simulink model "MCU_Input"  (R2022b)
settings: Solver=FixedStepDiscrete  StartTime=0.0  StopTime=10.0  FixedStep=1e-4  RelTol=1e-3
values from neighbouring files (symbols this model uses):
  C_ADC_Acc1Offset_i32 = 0.0    [MCU_Input_Sldd.sldd]    (also in MCU_Input_Sldd_objects.m = myPackage.Parameter)
  C_ADC_BrakeOffset_i32 = 0.0    [MCU_Input_Sldd.sldd]    (also in MCU_Input_Sldd_objects.m = myPackage.Parameter)
  C_ADC_HSTempGain_f32 = 0.0    [MCU_Input_Sldd.sldd]    (also in MCU_Input_Sldd_objects.m = myPackage.Parameter)
  C_ADC_HSTempOffset_i32 = 0.0    [MCU_Input_Sldd.sldd]    (also in MCU_Input_Sldd_objects.m = myPackage.Parameter)
  C_ADC_IdcOffset_i32 = 0.0    [MCU_Input_Sldd.sldd]    (also in MCU_Input_Sldd_objects.m = myPackage.Parameter)
  C_ADC_IGBTTable_i16 = 0.0    [MCU_Input_Sldd.sldd]    (also in MCU_Input_Sldd_objects.m = myPackage.Parameter)
  C_ADC_IGBTTempGain_f32 = 0.0    [MCU_Input_Sldd.sldd]    (also in MCU_Input_Sldd_objects.m = myPackage.Parameter)
  C_ADC_IGBTTempOffset_i32 = 0.0    [MCU_Input_Sldd.sldd]    (also in MCU_Input_Sldd_objects.m = myPackage.Parameter)
  C_ADC_MotorTemp1Gain_f32 = 0.0    [MCU_Input_Sldd.sldd]    (also in MCU_Input_Sldd_objects.m = myPackage.Parameter)
  C_ADC_MotorTemp1Offset_i32 = 0.0    [MCU_Input_Sldd.sldd]    (also in MCU_Input_Sldd_objects.m = myPackage.Parameter)
  C_ADC_MotorTempTable_i16 = 0.0    [MCU_Input_Sldd.sldd]    (also in MCU_Input_Sldd_objects.m = myPackage.Parameter)
  C_ADC_P12VOffset_i32 = 0.0    [MCU_Input_Sldd.sldd]    (also in MCU_Input_Sldd_objects.m = myPackage.Parameter)
  C_ADC_P15VOffset_i32 = 0.0    [MCU_Input_Sldd.sldd]    (also in MCU_Input_Sldd_objects.m = myPackage.Parameter)
  C_ADC_P5VOffset_i32 = 0.0    [MCU_Input_Sldd.sldd]    (also in MCU_Input_Sldd_objects.m = myPackage.Parameter)
  C_DCCurrent_DrvCoeff_f32 = 0.0    [MCU_Input_Sldd.sldd]    (also in MCU_Input_Sldd_objects.m = myPackage.Parameter)
  C_DCCurrent_GenCoeff_f32 = 0.0    [MCU_Input_Sldd.sldd]    (also in MCU_Input_Sldd_objects.m = myPackage.Parameter)
  C_Encoder_CurrentAdder_f32 = 0.0    [MCU_Input_Sldd.sldd]    (also in MCU_Input_Sldd_objects.m = myPackage.Parameter)
  C_Encoder_WaitTime_f32 = 0.0    [MCU_Input_Sldd.sldd]    (also in MCU_Input_Sldd_objects.m = myPackage.Parameter)
  C_Input_EncErr_u8 = 0.0    [MCU_Input_Sldd.sldd]    (also in MCU_Input_Sldd_objects.m = myPackage.Parameter)
  C_Rotate_RotateBits_u8 = 0.0    [MCU_Input_Sldd.sldd]    (also in MCU_Input_Sldd_objects.m = myPackage.Parameter)
  C_Rotate_SetAngle_u16 = 0.0    [MCU_Input_Sldd.sldd]    (also in MCU_Input_Sldd_objects.m = myPackage.Parameter)
  C_Rotate_SetAngleFlg_u8 = 0.0    [MCU_Input_Sldd.sldd]    (also in MCU_Input_Sldd_objects.m = myPackage.Parameter)
  C_SelfCheck_AvgCntSet_u16 = 0.0    [MCU_Input_Sldd.sldd]    (also in MCU_Input_Sldd_objects.m = myPackage.Parameter)
  C_SelfCheck_DelayTimeSet_u16 = 0.0    [MCU_Input_Sldd.sldd]    (also in MCU_Input_Sldd_objects.m = myPackage.Parameter)
  C_SelfCheck_IaoffsetDownLimt_u16 = 0.0    [MCU_Input_Sldd.sldd]    (also in MCU_Input_Sldd_objects.m = myPackage.Parameter)
  C_SelfCheck_IaoffsetUpLimt_u16 = 0.0    [MCU_Input_Sldd.sldd]    (also in MCU_Input_Sldd_objects.m = myPackage.Parameter)
  C_SelfCheck_IboffsetDownLimt_u16 = 0.0    [MCU_Input_Sldd.sldd]    (also in MCU_Input_Sldd_objects.m = myPackage.Parameter)
  C_SelfCheck_IboffsetUpLimt_u16 = 0.0    [MCU_Input_Sldd.sldd]    (also in MCU_Input_Sldd_objects.m = myPackage.Parameter)
  C_SelfCheck_IcoffsetDownLimt_u16 = 0.0    [MCU_Input_Sldd.sldd]    (also in MCU_Input_Sldd_objects.m = myPackage.Parameter)
  C_SelfCheck_IcoffsetUpLimt_u16 = 0.0    [MCU_Input_Sldd.sldd]    (also in MCU_Input_Sldd_objects.m = myPackage.Parameter)
  C_SelfCheck_OffsetUnCal_u8 = 0.0    [MCU_Input_Sldd.sldd]    (also in MCU_Input_Sldd_objects.m = myPackage.Parameter)
undefined symbols (not defined in the file or in its folder): AB_SAMPLE, ABC_SAMPLE, AC_SAMPLE, ANALOG, BC_SAMPLE, cAgeingMode, cParaRecogMode, cVvvfOpenMode, ParamCfg_AdAcc1K_u16, ParamCfg_AdBrakeK_u16, ParamCfg_AdIaK_u16, ParamCfg_AdIbK_u16, ParamCfg_AdIcK_u16, ParamCfg_AdKeyK_u16, ParamCfg_AdP12vK_u16, ParamCfg_AdP15vK_u16, ParamCfg_AdP5vK_u16, ParamCfg_AdUdcK_u16, ParamCfg_AdVonK_u16, ParamCfg_Avgcnt_u16, ParamCfg_BaseCur_u16, ParamCfg_BaseUdc_u16, ParamCfg_CommandSource_u16, ParamCfg_MaxSpeed_u16, ParamCfg_MotorNp_u16, ParamCfg_PosInit_u16, ParamCfg_PowerMax_u16, ParamCfg_PwmFreqLow_u16, ParamCfg_RotateDir_u16, ParamCfg_RotateNp_u16, ParamCfg_SampleMode_u16, ParamCfg_SensorSpeed_u16, ParamCfg_SmoPllKi_u16, ParamCfg_SmoPllKp_u16, ParamCfg_Stage_u16, ParamCfg_ThetaGain_u16, ParamCfg_UdcDefValue_u16, POWER_ON, STANDBY
libraries: simulink x41, YS_UserDefined_Library x4
(part 2 of 5)

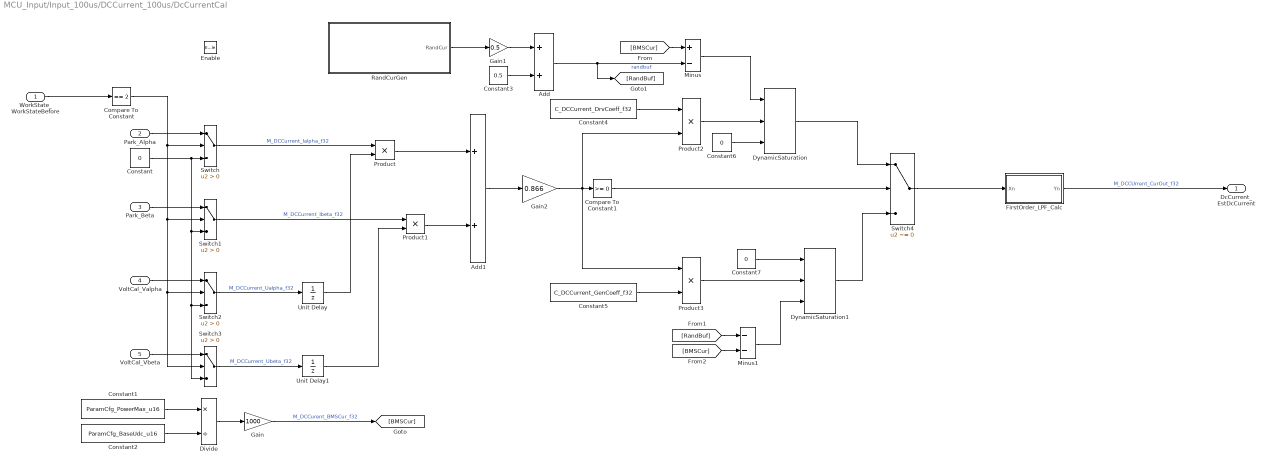
== system MCU_Input/Input_100us/DCCurrent_100us/DcCurrentCal ==
  WorkState_WorkStateBefore : Inport
  Park_Alpha : Inport  Port=2
  Park_Beta : Inport  Port=3
  VoltCal_Valpha : Inport  Port=4
  VoltCal_Vbeta : Inport  Port=5
  Enable : EnablePort
  Add : Sum
  Add1 : Sum
  Compare To Constant : simulink/Logic and Bit Operations/Compare To Constant  relop===  const=2  OutDataTypeStr=boolean
  Compare To Constant1 : simulink/Logic and Bit Operations/Compare To Constant  relop=>=  const=0  OutDataTypeStr=boolean
  Constant : Constant  Value=0  OutDataTypeStr=single
  Constant1 : Constant  Value=ParamCfg_PowerMax_u16
  Constant2 : Constant  Value=ParamCfg_BaseUdc_u16
  Constant3 : Constant  Value=0.5  OutDataTypeStr=single
  Constant4 : Constant  Value=C_DCCurrent_DrvCoeff_f32
  Constant5 : Constant  Value=C_DCCurrent_GenCoeff_f32
  Constant6 : Constant  Value=0  OutDataTypeStr=single
  Constant7 : Constant  Value=0  OutDataTypeStr=single
  Divide : Product  Inputs=*/
  DynamicSaturation : YS_UserDefined_Library/Saturation/DynamicSaturation
      settings: SourceProductName=YS
  DynamicSaturation1 : YS_UserDefined_Library/Saturation/DynamicSaturation
      settings: SourceProductName=YS
  FirstOrder_LPF_Calc : Subsystem
  Gain : Gain  Gain=1000  OutDataTypeStr=single
  Gain1 : Gain  Gain=0.5  OutDataTypeStr=single
  Gain2 : Gain  Gain=0.866
  Minus : Sum  Inputs=+-
  Minus1 : Sum  Inputs=--
  Product{,1..3} (4 alike) : Product
  RandCurGen : Subsystem
  Switch{,1..3} (4 alike) : Switch  Criteria=u2 > Threshold  SaturateOnIntegerOverflow=off  InputSameDT=off
  Switch4 : Switch  Criteria=u2 ~= 0  SaturateOnIntegerOverflow=off  InputSameDT=off
  Unit Delay : UnitDelay  SampleTime=-1  HasFrameUpgradeWarning=on
  Unit Delay1 : UnitDelay  SampleTime=-1  HasFrameUpgradeWarning=on
  DcCurrent_EstDcCurrent : Outport
  wires:
  WorkState_WorkStateBefore/1 -> Compare To Constant/1
  Constant/1 -> Switch3/3, Switch2/3, Switch1/3, Switch/3
  Compare To Constant/1 -> Switch3/2, Switch2/2, Switch1/2, Switch/2
  VoltCal_Vbeta/1 -> Switch3/1
  VoltCal_Valpha/1 -> Switch2/1
  Park_Alpha/1 -> Switch/1
  Park_Beta/1 -> Switch1/1
  Switch/1 -> Product/1  "M_DCCurrent_Ialpha_f32"
  Switch1/1 -> Product1/1  "M_DCCurrent_Ibeta_f32"
  Switch2/1 -> Unit Delay/1  "M_DCCurrent_Ualpha_f32"
  Switch3/1 -> Unit Delay1/1  "M_DCCurrent_Ubeta_f32"
  Constant1/1 -> Divide/1
  Constant2/1 -> Divide/2
  Divide/1 -> Gain/1
  Gain/1 -> [BMSCur]  "M_DCCurent_BMSCur_f32"
  RandCurGen/1(RandCur) -> Gain1/1
  Gain1/1 -> Add/1
  Constant3/1 -> Add/2
  Add/1 -> [RandBuf], Minus/2  "randbuf"
  Unit Delay/1 -> Product/2
  Unit Delay1/1 -> Product1/2
  Product/1 -> Add1/1
  Product1/1 -> Add1/2
  Add1/1 -> Gain2/1
  Gain2/1 -> Product2/2, Product3/1, Compare To Constant1/1
  Compare To Constant1/1 -> Switch4/2
  Constant4/1 -> Product2/1
  Product2/1 -> DynamicSaturation/2
  Constant6/1 -> DynamicSaturation/3
  [BMSCur] -> Minus/1
  Minus/1 -> DynamicSaturation/1
  DynamicSaturation/1 -> Switch4/1
  Constant5/1 -> Product3/2
  Product3/1 -> DynamicSaturation1/2
  Minus1/1 -> DynamicSaturation1/3
  [BMSCur] -> Minus1/2
  [RandBuf] -> Minus1/1
  Constant7/1 -> DynamicSaturation1/1
  DynamicSaturation1/1 -> Switch4/3
  Switch4/1 -> FirstOrder_LPF_Calc/1(Xn)
  FirstOrder_LPF_Calc/1(Yn) -> DcCurrent_EstDcCurrent/1  "M_DCCUrrent_CurOut_f32"

== system MCU_Input/Input_100us/ETheta/En ==
  note: 旋变零位标定
  Rotate_PosNew : Inport
  Rotate_PosDelt : Inport  Port=2
  Enable : EnablePort
  Constant : Constant  Value=C_Encoder_CurrentAdder_f32  OutDataTypeStr=single
  Constant1 : Constant  Value=4800  OutDataTypeStr=single
  Constant2 : Constant  Value=ParamCfg_PwmFreqLow_u16  OutDataTypeStr=uint16
  Constant3 : Constant  Value=0.28  OutDataTypeStr=single
  Constant4 : Constant  Value=C_Encoder_WaitTime_f32
  Constant5 : Constant  Value=ParamCfg_BaseCur_u16  OutDataTypeStr=uint16
  Divide : Product  Inputs=*/
  EncMode_Calc : Stateflow chart  TreatAsAtomicUnit=on
  Product : Product
  Product1 : Product
  Product2 : Product
  Sqrt(2) : Constant  Value=1.414213562373  OutDataTypeStr=single
  EAngle : Outport
  CurrentOutput : Outport  Port=2
  ZeroP : Outport  Port=3
  OverFlg : Outport  Port=4
  CurOut : Outport  Port=5
  wires:
  Constant2/1 -> Product1/1, Divide/2  "ActFrq"
  Constant/1 -> Product/1
  Product/1 -> Divide/1
  Rotate_PosNew/1 -> EncMode_Calc/3(PosInput)
  Divide/1 -> EncMode_Calc/1(CurAdder)
  Constant1/1 -> Product/2
  Rotate_PosDelt/1 -> EncMode_Calc/4(PosDelt)
  Constant3/1 -> EncMode_Calc/2(GivenCurrent)
  EncMode_Calc/1(EAngle) -> EAngle/1
  EncMode_Calc/2(CurrentOutput) -> CurrentOutput/1
  Constant4/1 -> Product1/2
  Product1/1 -> EncMode_Calc/5(WaitTimeOut)
  Constant5/1 -> Product2/1
  Sqrt(2)/1 -> Product2/2
  Product2/1 -> EncMode_Calc/6(Idn)
  EncMode_Calc/3(ZeroP) -> ZeroP/1
  EncMode_Calc/4(OverFlg) -> OverFlg/1
  EncMode_Calc/5(CurOut) -> CurOut/1

== system MCU_Input/Input_100us/ETheta1/En ==
  note: 旋变零位标定
  cParaRecogMode : Inport
  Rotate_PosNew : Inport  Port=2
  Rotate_PosDelt : Inport  Port=3
  Standby : Inport  Port=4
  Constant : Constant  Value=C_Encoder_CurrentAdder_f32  OutDataTypeStr=single
  Constant1 : Constant  Value=4800  OutDataTypeStr=single
  Constant2 : Constant  Value=ParamCfg_PwmFreqLow_u16  OutDataTypeStr=uint16
  Constant3 : Constant  Value=0.28  OutDataTypeStr=single
  Constant4 : Constant  Value=C_Encoder_WaitTime_f32
  Constant5 : Constant  Value=ParamCfg_BaseCur_u16  OutDataTypeStr=uint16
  Divide : Product  Inputs=*/
  EncMode_Calc : Stateflow chart  TreatAsAtomicUnit=on
  Product : Product
  Product1 : Product
  Product2 : Product
  Sqrt(2) : Constant  Value=1.414213562373  OutDataTypeStr=single
  EAngle : Outport
  CurrentOutput : Outport  Port=2
  ZeroP : Outport  Port=3
  OverFlg : Outport  Port=4
  CurOut : Outport  Port=5
  wires:
  Constant2/1 -> Product1/1, Divide/2  "ActFrq"
  Constant/1 -> Product/1
  Product/1 -> Divide/1
  Rotate_PosNew/1 -> EncMode_Calc/4(Rotate_PosNew)
  Divide/1 -> EncMode_Calc/1(CurAdder)
  Constant1/1 -> Product/2
  Rotate_PosDelt/1 -> EncMode_Calc/5(Rotate_PosDelt)
  Constant3/1 -> EncMode_Calc/2(GivenCurrent)
  EncMode_Calc/1(EAngle) -> EAngle/1
  EncMode_Calc/2(CurrentOutput) -> CurrentOutput/1
  Constant4/1 -> Product1/2
  Product1/1 -> EncMode_Calc/7(WaitTimeOut)
  Constant5/1 -> Product2/1
  Sqrt(2)/1 -> Product2/2
  Product2/1 -> EncMode_Calc/8(Idn)
  EncMode_Calc/3(ZeroP) -> ZeroP/1
  EncMode_Calc/4(OverFlg) -> OverFlg/1
  EncMode_Calc/5(CurOut) -> CurOut/1
  cParaRecogMode/1 -> EncMode_Calc/3(ParaRecogMode)
  Standby/1 -> EncMode_Calc/6(Standby)

== system MCU_Input/Input_100us/Encoder_100us/Encoder_100us ==
  note: 初始化操作可以完成
      | 1、SinAverage
      | 2、CosAverage
      | 3、SinAmplitude
      | 4、CosAmplitude
      |
      | 初始化无法完成：
      | 1、SinAmplitude_Inverse
      | 2、CosAmplitude_Inverse
  note: 保证可以被ParamCfg的参数写入
  Calib_Stage : Inport
  AvgCnt : Inport  Port=2
  CosDigitalValue : Inport  Port=3
  SinDigitalValue : Inport  Port=4
  PWMPrdChg_PWMFreq : Inport  Port=5
  Data Store Memory : DataStoreMemory  DataStoreName=SinMax  WriteAfterWriteMsg=warning  InitialValue=2048  ShowAdditionalParam=off
  Data Store Memory1 : DataStoreMemory  DataStoreName=SinAvg  WriteAfterWriteMsg=warning  InitialValue=ParamCfg_Sinavg_u16  ShowAdditionalParam=off  OutDataTypeStr=uint16  StateMustResolveToSignalObject=on
  Data Store Memory2 : DataStoreMemory  DataStoreName=SinAmp  WriteAfterWriteMsg=warning  InitialValue=ParamCfg_Sinamp_u16  ShowAdditionalParam=off  OutDataTypeStr=uint16  StateMustResolveToSignalObject=on
  Data Store Memory3 : DataStoreMemory  DataStoreName=CosAvg  WriteAfterWriteMsg=warning  InitialValue=ParamCfg_Cosavg_u16  ShowAdditionalParam=off  OutDataTypeStr=uint16  StateMustResolveToSignalObject=on
  Data Store Memory4 : DataStoreMemory  DataStoreName=CosAmp  WriteAfterWriteMsg=warning  InitialValue=ParamCfg_Cosamp_u16  ShowAdditionalParam=off  OutDataTypeStr=uint16  StateMustResolveToSignalObject=on
  Data Store Memory5 : DataStoreMemory  DataStoreName=CosMax  WriteAfterWriteMsg=warning  InitialValue=2048  ShowAdditionalParam=off
  Data Store Memory6 : DataStoreMemory  DataStoreName=SinMin  WriteAfterWriteMsg=warning  InitialValue=2048  ShowAdditionalParam=off
  Data Store Memory7 : DataStoreMemory  DataStoreName=CosMin  WriteAfterWriteMsg=warning  InitialValue=2048  ShowAdditionalParam=off
  EncAngleCal : Subsystem  TreatAsAtomicUnit=on
      settings: RTWSystemCode=Nonreusable function
  EncCalibCal : Stateflow chart  TreatAsAtomicUnit=on
      settings: RTWSystemCode=Nonreusable function
  EncCalibCal1 : Stateflow chart  Commented=on  TreatAsAtomicUnit=on
      settings: RTWSystemCode=Nonreusable function
  EncCalibCal2 : Stateflow chart  Commented=on  TreatAsAtomicUnit=on
      settings: RTWSystemCode=Nonreusable function
  CosAverage : Outport
  SinAverage : Outport  Port=2
  EncCal_Angle : Outport  Port=3
  wires:
  CosDigitalValue/1 -> EncCalibCal/3(CosDigitalValue)
  EncCalibCal/1(CosValue) -> EncAngleCal/1(CosValue), CosAverage/1
  SinDigitalValue/1 -> EncCalibCal/4(SinDigitalValue)
  Calib_Stage/1 -> EncCalibCal/1(Calib_Stage)
  EncCalibCal/2(SinValue) -> EncAngleCal/2(SinValue), SinAverage/1
  AvgCnt/1 -> EncCalibCal/2(AvgCnt)
  EncAngleCal/1(EncCal_Angle) -> EncCal_Angle/1
  PWMPrdChg_PWMFreq/1 -> EncAngleCal/3(PWMPrdChg_PWMFreq)

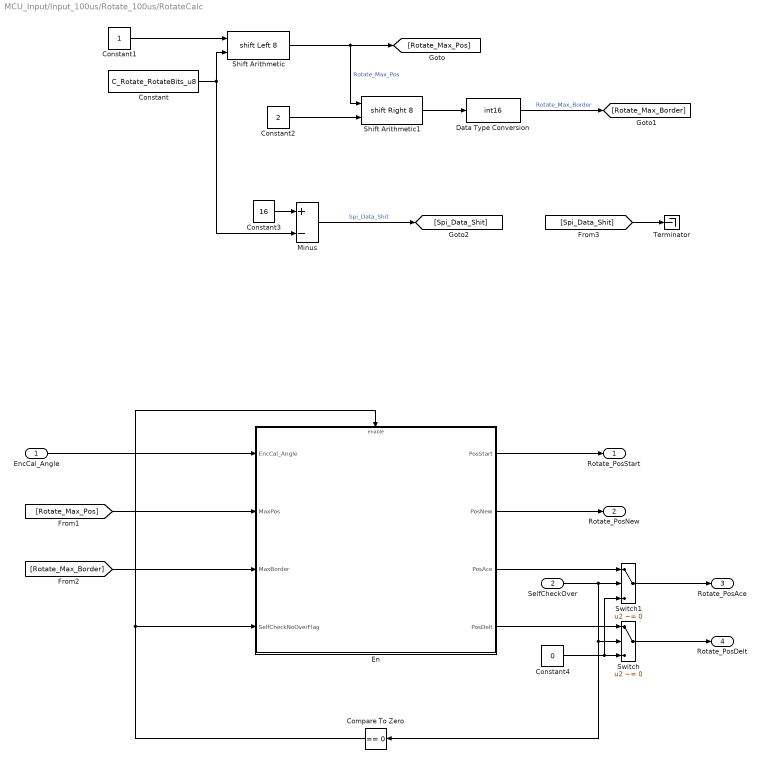
== system MCU_Input/Input_100us/Rotate_100us/RotateCalc ==
  EncCal_Angle : Inport
  SelfCheckOver : Inport  Port=2
  Compare To Zero : simulink/Logic and Bit Operations/Compare To Zero  relop===  OutDataTypeStr=boolean
  Constant : Constant  Value=C_Rotate_RotateBits_u8
  Constant1 : Constant  OutDataTypeStr=uint16
  Constant2 : Constant  Value=2  OutDataTypeStr=uint8
  Constant3 : Constant  Value=16  OutDataTypeStr=uint16
  Constant4 : Constant  Value=0  OutDataTypeStr=int16
  Data Type Conversion : DataTypeConversion  OutDataTypeStr=int16  SaturateOnIntegerOverflow=off  RndMeth=Floor
  En : Subsystem
  Minus : Sum  Inputs=+-
  Shift Arithmetic : ArithShift  BitShiftNumberSource=Input port  BitShiftNumber=8  BitShiftDirection=Left
      settings: InputPortMap=u0,p1
  Shift Arithmetic1 : ArithShift  BitShiftNumberSource=Input port  BitShiftNumber=8  BitShiftDirection=Right
      settings: InputPortMap=u0,p1
  Switch : Switch  Criteria=u2 ~= 0  SaturateOnIntegerOverflow=off  InputSameDT=off
  Switch1 : Switch  Criteria=u2 ~= 0  SaturateOnIntegerOverflow=off  InputSameDT=off
  Terminator : Terminator
  Rotate_PosStart : Outport
  Rotate_PosNew : Outport  Port=2
  Rotate_PosAce : Outport  Port=3
  Rotate_PosDelt : Outport  Port=4
  wires:
  Shift Arithmetic/1 -> Shift Arithmetic1/1, [Rotate_Max_Pos]  "Rotate_Max_Pos"
  Constant3/1 -> Minus/1
  Constant/1 -> Shift Arithmetic/2, Minus/2
  Minus/1 -> [Spi_Data_Shit]  "Spi_Data_Shit"
  Data Type Conversion/1 -> [Rotate_Max_Border]  "Rotate_Max_Border"
  Constant1/1 -> Shift Arithmetic/1
  Constant2/1 -> Shift Arithmetic1/2
  Shift Arithmetic1/1 -> Data Type Conversion/1
  [Spi_Data_Shit] -> Terminator/1
  SelfCheckOver/1 -> Switch1/2, Compare To Zero/1, Switch/2
  Switch/1 -> Rotate_PosDelt/1
  Constant4/1 -> Switch1/3, Switch/3
  Switch1/1 -> Rotate_PosAce/1
  EncCal_Angle/1 -> En/1(EncCal_Angle)
  [Rotate_Max_Pos] -> En/2(MaxPos)
  [Rotate_Max_Border] -> En/3(MaxBorder)
  Compare To Zero/1 -> En/Enable, En/4(SelfCheckNoOverFlag)
  En/1(PosStart) -> Rotate_PosStart/1
  En/4(PosDelt) -> Switch/1
  En/2(PosNew) -> Rotate_PosNew/1
  En/3(PosAce) -> Switch1/1

== system MCU_Input/Input_100us/SelfCheck_100us/EnCal ==
  note: POWERON
  note: 保证再STANDBY状态下，满足条件会一直出发零漂检测
  SpeedCal_Speed20msABS : Inport
  WorkState_IgbtWorkFlag : Inport  Port=2
  StanbyState : Inport  Port=3
  PoweronState : Inport  Port=4
  OffsetCalOverFlg : Inport  Port=5
  Compare To Constant1 : simulink/Logic and Bit Operations/Compare To Constant  relop=<  const=50  OutDataTypeStr=uint8
  Compare To Zero : simulink/Logic and Bit Operations/Compare To Zero  relop===  OutDataTypeStr=uint8
  Constant2 : Constant  OutDataTypeStr=uint8
  Constant3 : Constant  Value=0  OutDataTypeStr=uint8
  Data Type Conversion2 : DataTypeConversion  OutDataTypeStr=uint8  SaturateOnIntegerOverflow=off  RndMeth=Floor
  Logical Operator : Logic  Inputs=3  AllPortsSameDT=off  OutDataTypeStr=boolean
  Logical Operator1 : Logic  Operator=NOT  AllPortsSameDT=off  OutDataTypeStr=boolean
  Switch : Switch  Criteria=u2 ~= 0  SaturateOnIntegerOverflow=off  InputSameDT=off
  Switch1 : Switch  Criteria=u2 ~= 0  SaturateOnIntegerOverflow=off  InputSameDT=off
  Unit Delay : UnitDelay  SampleTime=-1  HasFrameUpgradeWarning=on
  M_Selfcheck_EnFlg_u8 : Outport
  wires:
  Constant3/1 -> Switch1/3
  Compare To Constant1/1 -> Logical Operator/1  "M_Selfcheck_SpeedEnFlg_u8"
  Logical Operator/1 -> Switch/2
  Constant2/1 -> Switch/1
  Compare To Zero/1 -> Logical Operator/2  "M_Selfcheck_IgbtWorkEnFlg_u8"
  SpeedCal_Speed20msABS/1 -> Compare To Constant1/1
  Data Type Conversion2/1 -> Switch1/1
  Unit Delay/1 -> Logical Operator1/1
  Logical Operator1/1 -> Data Type Conversion2/1
  Switch1/1 -> Switch/3
  Switch/1 -> M_Selfcheck_EnFlg_u8/1  "M_Selfcheck_EnFlg_u8"
  PoweronState/1 -> Switch1/2
  StanbyState/1 -> Logical Operator/3
  OffsetCalOverFlg/1 -> Unit Delay/1
  WorkState_IgbtWorkFlag/1 -> Compare To Zero/1

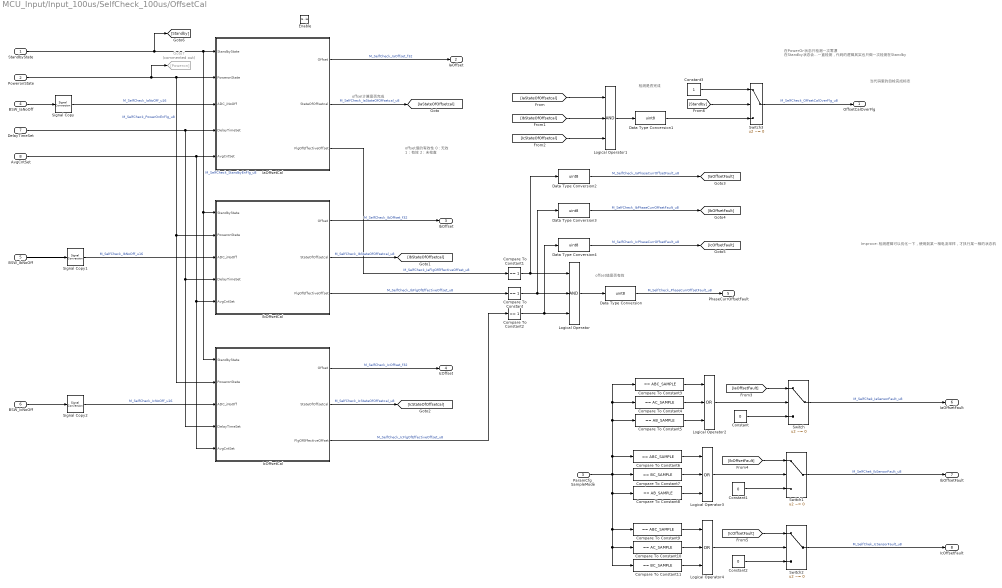
== system MCU_Input/Input_100us/SelfCheck_100us/OffsetCal ==
  note: Improve:
      | 检测逻辑可以优化一下，使用到某一相电流采样，才执行某一相的状态机
  note: 在PowerOn状态只检测一次零漂
      | 在Standby状态会一直检测，代码的逻辑其实也只做一次检测在Standby
  note: 当代码里的自检完成标志
  note: offset值是否有效
  note: 检测是否完成
  note: offset值的有效性
      | 0：无效
      | 1：有效
      | 2：未检查
  note: offset计算是否完成
  StandbyState : Inport
  PoweronState : Inport  Port=2
  ParamCfg_SampleMode : Inport  Port=3
  BSW_IaNoOff : Inport  Port=4
  BSW_IbNoOff : Inport  Port=5
  BSW_IcNoOff : Inport  Port=6
  DelayTimeSet : Inport  Port=7
  AvgCntSet : Inport  Port=8
  Enable : EnablePort
  Compare To Constant : simulink/Logic and Bit Operations/Compare To Constant  relop===  const=1  OutDataTypeStr=boolean
  Compare To Constant1 : simulink/Logic and Bit Operations/Compare To Constant  relop===  const=1  OutDataTypeStr=boolean
  Compare To Constant10 : simulink/Logic and Bit Operations/Compare To Constant  relop===  const=AC_SAMPLE  OutDataTypeStr=boolean
  Compare To Constant11 : simulink/Logic and Bit Operations/Compare To Constant  relop===  const=BC_SAMPLE  OutDataTypeStr=boolean
  Compare To Constant2 : simulink/Logic and Bit Operations/Compare To Constant  relop===  const=1  OutDataTypeStr=boolean
  Compare To Constant3 : simulink/Logic and Bit Operations/Compare To Constant  relop===  const=ABC_SAMPLE  OutDataTypeStr=boolean
  Compare To Constant4 : simulink/Logic and Bit Operations/Compare To Constant  relop===  const=AC_SAMPLE  OutDataTypeStr=boolean
  Compare To Constant5 : simulink/Logic and Bit Operations/Compare To Constant  relop===  const=AB_SAMPLE  OutDataTypeStr=boolean
  Compare To Constant6 : simulink/Logic and Bit Operations/Compare To Constant  relop===  const=ABC_SAMPLE  OutDataTypeStr=boolean
  Compare To Constant7 : simulink/Logic and Bit Operations/Compare To Constant  relop===  const=BC_SAMPLE  OutDataTypeStr=boolean
  Compare To Constant8 : simulink/Logic and Bit Operations/Compare To Constant  relop===  const=AB_SAMPLE  OutDataTypeStr=boolean
  Compare To Constant9 : simulink/Logic and Bit Operations/Compare To Constant  relop===  const=ABC_SAMPLE  OutDataTypeStr=boolean
  Constant : Constant  Value=0  OutDataTypeStr=uint8
  Constant1 : Constant  Value=0  OutDataTypeStr=uint8
  Constant2 : Constant  Value=0  OutDataTypeStr=uint8
  Constant3 : Constant  OutDataTypeStr=uint8
  Data Type Conversion{,1..4} (5 alike) : DataTypeConversion  OutDataTypeStr=uint8  SaturateOnIntegerOverflow=off  RndMeth=Floor
  Goto7 : Goto  Commented=on  GotoTag=Poweron
  IaOffsetCal : Stateflow chart  TreatAsAtomicUnit=on
  IbOffsetCal : Stateflow chart  TreatAsAtomicUnit=on
  IcOffsetCal : Stateflow chart  TreatAsAtomicUnit=on
  Logical Operator : Logic  Inputs=3  AllPortsSameDT=off  OutDataTypeStr=boolean
  Logical Operator1 : Logic  Inputs=3  AllPortsSameDT=off  OutDataTypeStr=boolean
  Logical Operator2 : Logic  Operator=OR  Inputs=3  AllPortsSameDT=off  OutDataTypeStr=boolean
  Logical Operator3 : Logic  Operator=OR  Inputs=3  AllPortsSameDT=off  OutDataTypeStr=boolean
  Logical Operator4 : Logic  Operator=OR  Inputs=3  AllPortsSameDT=off  OutDataTypeStr=boolean
  Signal Copy : SignalConversion  OverrideOpt=off
  Signal Copy1 : SignalConversion  OverrideOpt=off
  Signal Copy2 : SignalConversion  OverrideOpt=off
  Switch{,1..3} (4 alike) : Switch  Criteria=u2 ~= 0  SaturateOnIntegerOverflow=off  InputSameDT=off
  OffsetCalOverFlg : Outport
  IaOffset : Outport  Port=2
  IbOffset : Outport  Port=3
  IcOffset : Outport  Port=4
  PhaseCurrOffsetFault : Outport  Port=5
  IaOffsetFault : Outport  Port=6
  IbOffsetFault : Outport  Port=7
  IcOffsetFault : Outport  Port=8
  wires:
  BSW_IaNoOff/1 -> Signal Copy/1
  BSW_IbNoOff/1 -> Signal Copy1/1
  BSW_IcNoOff/1 -> Signal Copy2/1
  IaOffsetCal/1(Offset) -> IaOffset/1  "M_SelfCheck_IaOffset_f32"
  PoweronState/1 -> Goto7/1, IcOffsetCal/2(PoweronState), IbOffsetCal/2(PoweronState), IaOffsetCal/2(PoweronState)  "M_SelfCheck_PowerOnEnFlg_u8"
  IaOffsetCal/2(StateOfOffsetcal) -> [IaStateOfOffsetcal]  "M_SelfCheck_IaStateOfOffsetcal_u8"
  IaOffsetCal/3(FlgOfEffectiveOffset) -> Compare To Constant1/1  "M_SelfCheck_IaFlgOfEffectiveOffset_u8"
  IbOffsetCal/1(Offset) -> IbOffset/1  "M_SelfCheck_IbOffset_f32"
  IbOffsetCal/2(StateOfOffsetcal) -> [IbStateOfOffsetcal]  "M_SelfCheck_IbStateOfOffsetcal_u8"
  IbOffsetCal/3(FlgOfEffectiveOffset) -> Compare To Constant/1  "M_SelfCheck_IbFlgOfEffectiveOffset_u8"
  IcOffsetCal/1(Offset) -> IcOffset/1  "M_SelfCheck_IcOffset_f32"
  IcOffsetCal/2(StateOfOffsetcal) -> [IcStateOfOffsetcal]  "M_SelfCheck_IcStateOfOffsetcal_u8"
  IcOffsetCal/3(FlgOfEffectiveOffset) -> Compare To Constant2/1  "M_SelfCheck_IcFlgOfEffectiveOffset_u8"
  Logical Operator/1 -> Data Type Conversion/1
  Data Type Conversion/1 -> PhaseCurrOffsetFault/1  "M_SelfCheck_PhaseCurrOffsetFault_u8"
  [IbStateOfOffsetcal] -> Logical Operator1/2
  [IaStateOfOffsetcal] -> Logical Operator1/1
  [IcStateOfOffsetcal] -> Logical Operator1/3
  Logical Operator1/1 -> Data Type Conversion1/1
  Switch3/1 -> OffsetCalOverFlg/1  "M_SelfCheck_OffsetCalOverFlg_u8"
  Compare To Constant1/1 -> Data Type Conversion2/1, Logical Operator/1
  Compare To Constant/1 -> Logical Operator/2, Data Type Conversion3/1
  Compare To Constant2/1 -> Logical Operator/3, Data Type Conversion4/1
  Data Type Conversion2/1 -> [IaOffsetFault]  "M_SelfCheck_IaPhaseCurrOffsetFault_u8"
  Data Type Conversion3/1 -> [IbOffsetFault]  "M_SelfCheck_IbPhaseCurrOffsetFault_u8"
  Data Type Conversion4/1 -> [IcOffsetFault]  "M_SelfCheck_IcPhaseCurrOffsetFault_u8"
  StandbyState/1 -> [Standby], IaOffsetCal/1(StandbyState), IcOffsetCal/1(StandbyState), IbOffsetCal/1(StandbyState)  "M_SelfCheck_StandbyEnFlg_u8"
  ParamCfg_SampleMode/1 -> Compare To Constant3/1, Compare To Constant4/1, Compare To Constant5/1, Compare To Constant6/1, Compare To Constant11/1, Compare To Constant10/1, Compare To Constant9/1, Compare To Constant8/1, Compare To Constant7/1
  Compare To Constant4/1 -> Logical Operator2/2
  Compare To Constant3/1 -> Logical Operator2/1
  Compare To Constant5/1 -> Logical Operator2/3
  Logical Operator2/1 -> Switch/2
  [IaOffsetFault] -> Switch/1
  Constant/1 -> Switch/3
  Switch/1 -> IaOffsetFault/1  "M_SelfChek_IaSensorFault_u8"
  Compare To Constant7/1 -> Logical Operator3/2
  Compare To Constant6/1 -> Logical Operator3/1
  Compare To Constant8/1 -> Logical Operator3/3
  Constant1/1 -> Switch1/3
  [IbOffsetFault] -> Switch1/1
  Logical Operator3/1 -> Switch1/2
  Compare To Constant10/1 -> Logical Operator4/2
  Compare To Constant9/1 -> Logical Operator4/1
  Compare To Constant11/1 -> Logical Operator4/3
  Constant2/1 -> Switch2/3
  [IcOffsetFault] -> Switch2/1
  Logical Operator4/1 -> Switch2/2
  Switch1/1 -> IbOffsetFault/1  "M_SelfChek_IbSensorFault_u8"
  Switch2/1 -> IcOffsetFault/1  "M_SelfChek_IcSensorFault_u8"
  [Standby] -> Switch3/2
  Constant3/1 -> Switch3/1
  Data Type Conversion1/1 -> Switch3/3
  Signal Copy/1 -> IaOffsetCal/3(ADC_iNoOff)  "M_SelfCheck_IaNoOff_u16"
  AvgCntSet/1 -> IcOffsetCal/5(AvgCntSet), IbOffsetCal/5(AvgCntSet), IaOffsetCal/5(AvgCntSet)
  DelayTimeSet/1 -> IcOffsetCal/4(DelayTimeSet), IbOffsetCal/4(DelayTimeSet), IaOffsetCal/4(DelayTimeSet)
  Signal Copy1/1 -> IbOffsetCal/3(ADC_iNoOff)  "M_SelfCheck_IbNoOff_u16"
  Signal Copy2/1 -> IcOffsetCal/3(ADC_iNoOff)  "M_SelfCheck_IcNoOff_u16"

== system MCU_Input/Input_100us/ThetaCal_100us/If Action Subsystem ==
  PWMPrdChg_PWMPrd : Inport
  vvvfCtrl_FreqCmd : Inport  Port=2
  Action Port : ActionPort  ActionPortLabel=if(u1 == 1)
  Add : Sum
  Mapping : YS_UserDefined_Library/Others/Mapping
      settings: SourceProductName=YS
  Product : Product
  Unit Delay : UnitDelay  SampleTime=-1  HasFrameUpgradeWarning=on
  mTheta : Outport
  wires:
  PWMPrdChg_PWMPrd/1 -> Product/1
  vvvfCtrl_FreqCmd/1 -> Product/2
  Add/1 -> Mapping/1, Unit Delay/1
  Unit Delay/1 -> Add/2
  Product/1 -> Add/1
  Mapping/1 -> mTheta/1

== system MCU_Input/Input_100us/ThetaCal_100us/If Action Subsystem1 ==
  PWMPrdChg_PWMPrd : Inport
  vvvfCtrl_FreqCmd : Inport  Port=2
  Action Port : ActionPort  ActionPortLabel=elseif(u2==1)
  Add : Sum
  Mapping : YS_UserDefined_Library/Others/Mapping
      settings: SourceProductName=YS
  Product : Product
  Unit Delay : UnitDelay  SampleTime=-1  HasFrameUpgradeWarning=on
  mTheta : Outport
  wires:
  Mapping/1 -> mTheta/1
  Product/1 -> Add/1
  Unit Delay/1 -> Add/2
  Add/1 -> Unit Delay/1, Mapping/1
  vvvfCtrl_FreqCmd/1 -> Product/2
  PWMPrdChg_PWMPrd/1 -> Product/1

== system MCU_Input/Input_100us/ThetaCal_100us/If Action Subsystem2 ==
  note: 4096
  POSTheta : Inport
  Action Port : ActionPort  ActionPortLabel=else
  Constant : Constant  OutDataTypeStr=single
  Constant1 : Constant  Value=ParamCfg_MotorNp_u16
  Constant2 : Constant  Value=ParamCfg_RotateNp_u16
  Constant3 : Constant  OutDataTypeStr=single
  Constant5 : Constant  OutDataTypeStr=int16
  Constant6 : Constant  Value=12  OutDataTypeStr=uint8
  Divide : Product  Inputs=*/
  Divide1 : Product  Inputs=*/
  Product : Product
  Product1 : Product
  Rem : Math  Operator=rem
  Shift Arithmetic : ArithShift  BitShiftNumberSource=Input port  BitShiftNumber=8  BitShiftDirection=Left
      settings: InputPortMap=u0,p1
  mTheta : Outport
  tag scope: MaxPos=global
  wires:
  [MaxPos] -> Divide/2
  Constant/1 -> Divide/1
  POSTheta/1 -> Product/1
  Product/1 -> Product1/1
  Divide/1 -> Product/2
  Constant1/1 -> Divide1/1
  Constant2/1 -> Divide1/2
  Divide1/1 -> Product1/2  "motor_rotate_np_gain"
  Product1/1 -> Rem/1
  Constant3/1 -> Rem/2
  Rem/1 -> mTheta/1
  Constant5/1 -> Shift Arithmetic/1
  Shift Arithmetic/1 -> [MaxPos]
  Constant6/1 -> Shift Arithmetic/2

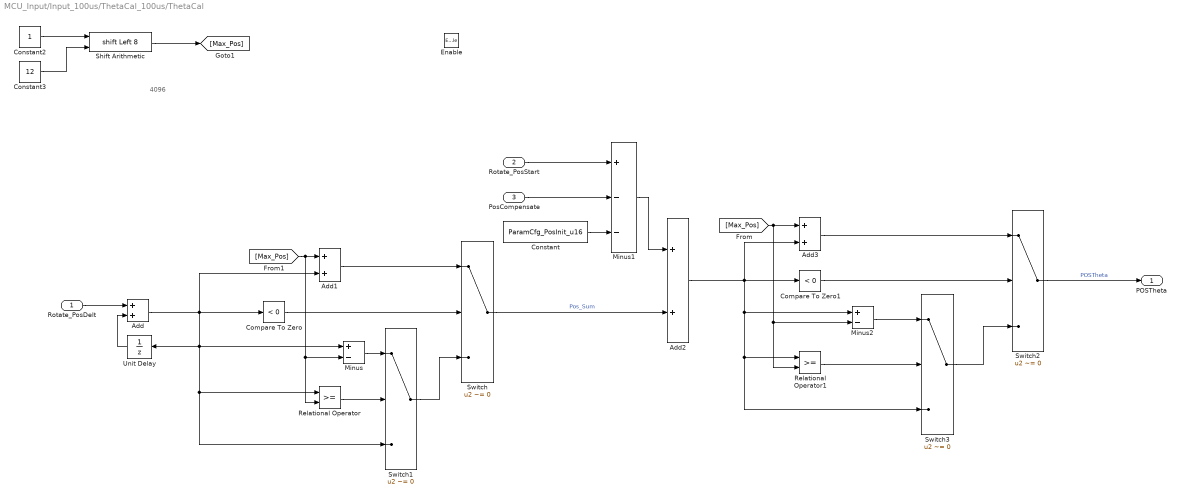
== system MCU_Input/Input_100us/ThetaCal_100us/ThetaCal ==
  note: 4096
  Rotate_PosDelt : Inport
  Rotate_PosStart : Inport  Port=2
  PosCompensate : Inport  Port=3
  Enable : EnablePort
  Add : Sum  OutDataTypeStr=single
  Add1 : Sum
  Add2 : Sum
  Add3 : Sum
  Compare To Zero : simulink/Logic and Bit Operations/Compare To Zero  relop=<  OutDataTypeStr=boolean
  Compare To Zero1 : simulink/Logic and Bit Operations/Compare To Zero  relop=<  OutDataTypeStr=boolean
  Constant : Constant  Value=ParamCfg_PosInit_u16
  Constant2 : Constant  OutDataTypeStr=int16
  Constant3 : Constant  Value=12  OutDataTypeStr=uint8
  Minus : Sum  Inputs=+-
  Minus1 : Sum  Inputs=+--
  Minus2 : Sum  Inputs=+-
  Relational Operator : RelationalOperator  OutDataTypeStr=boolean  RndMeth=Simplest  InputSameDT=off
  Relational Operator1 : RelationalOperator  OutDataTypeStr=boolean  RndMeth=Simplest  InputSameDT=off
  Shift Arithmetic : ArithShift  BitShiftNumberSource=Input port  BitShiftNumber=8  BitShiftDirection=Left
      settings: InputPortMap=u0,p1
  Switch{,1..3} (4 alike) : Switch  Criteria=u2 ~= 0  SaturateOnIntegerOverflow=off  InputSameDT=off
  Unit Delay : UnitDelay  SampleTime=-1  HasFrameUpgradeWarning=on
  POSTheta : Outport
  wires:
  Add/1 -> Relational Operator/1, Switch1/3, Minus/1, Unit Delay/1, Compare To Zero/1, Add1/2
  Unit Delay/1 -> Add/2
  Rotate_PosDelt/1 -> Add/1
  Compare To Zero/1 -> Switch/2
  Constant2/1 -> Shift Arithmetic/1
  Constant3/1 -> Shift Arithmetic/2
  Shift Arithmetic/1 -> [Max_Pos]
  Add1/1 -> Switch/1
  [Max_Pos] -> Minus/2, Relational Operator/2, Add1/1
  Relational Operator/1 -> Switch1/2
  Minus/1 -> Switch1/1
  Switch1/1 -> Switch/3
  Switch/1 -> Add2/2  "Pos_Sum"
  Rotate_PosStart/1 -> Minus1/1
  PosCompensate/1 -> Minus1/2
  Minus1/1 -> Add2/1
  Add2/1 -> Minus2/1, Switch3/3, Relational Operator1/1, Add3/2, Compare To Zero1/1
  Compare To Zero1/1 -> Switch2/2
  Add3/1 -> Switch2/1
  [Max_Pos] -> Minus2/2, Relational Operator1/2, Add3/1
  Relational Operator1/1 -> Switch3/2
  Switch3/1 -> Switch2/3
  Minus2/1 -> Switch3/1
  Switch2/1 -> POSTheta/1  "POSTheta"
  Constant/1 -> Minus1/3

== system MCU_Input/Input_100us/ThetaCal_100us/ThetaOffsetGain ==
  SpeedSensor : Inport
  SpeedCal_Speed20ms : Inport  Port=2
  Constant : Constant  Value=ParamCfg_ThetaGain_u16
  Constant1 : Constant  Value=-0.001  OutDataTypeStr=single
  Constant2 : Constant  Value=0.001  OutDataTypeStr=single
  Product : Product
  Product1 : Product  OutDataTypeStr=single
  Switch : Switch  Criteria=u2 ~= 0  SaturateOnIntegerOverflow=off  InputSameDT=off
  PosCompensate : Outport
  wires:
  SpeedCal_Speed20ms/1 -> Product1/2
  Constant/1 -> Product/1
  Constant1/1 -> Switch/1
  Product/1 -> Product1/1  "mTheta_Offset_Gain"
  SpeedSensor/1 -> Switch/2
  Switch/1 -> Product/2
  Constant2/1 -> Switch/3
  Product1/1 -> PosCompensate/1

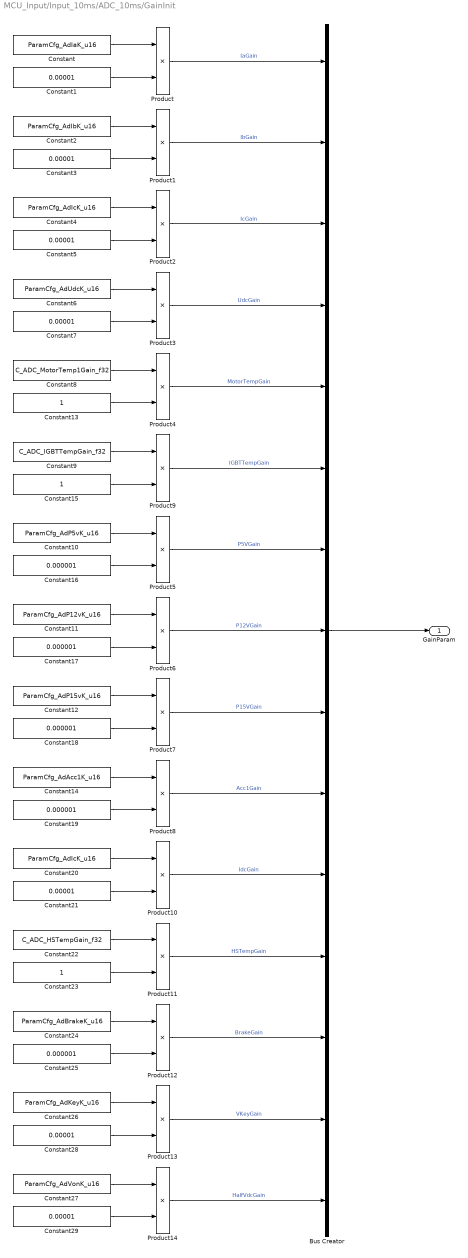
== system MCU_Input/Input_10ms/ADC_10ms/GainInit ==
  Bus Creator : BusCreator  Inputs=15
  Constant : Constant  Value=ParamCfg_AdIaK_u16
  Constant{1,3,5,7,21,28..29} (7 alike) : Constant  Value=0.00001  OutDataTypeStr=single
  Constant10 : Constant  Value=ParamCfg_AdP5vK_u16
  Constant11 : Constant  Value=ParamCfg_AdP12vK_u16
  Constant12 : Constant  Value=ParamCfg_AdP15vK_u16
  Constant13 : Constant  OutDataTypeStr=single
  Constant14 : Constant  Value=ParamCfg_AdAcc1K_u16
  Constant15 : Constant  OutDataTypeStr=single
  Constant{16..19,25} (5 alike) : Constant  Value=0.000001  OutDataTypeStr=single
  Constant2 : Constant  Value=ParamCfg_AdIbK_u16
  Constant20 : Constant  Value=ParamCfg_AdIcK_u16
  Constant22 : Constant  Value=C_ADC_HSTempGain_f32
  Constant23 : Constant  OutDataTypeStr=single
  Constant24 : Constant  Value=ParamCfg_AdBrakeK_u16
  Constant26 : Constant  Value=ParamCfg_AdKeyK_u16
  Constant27 : Constant  Value=ParamCfg_AdVonK_u16
  Constant4 : Constant  Value=ParamCfg_AdIcK_u16
  Constant6 : Constant  Value=ParamCfg_AdUdcK_u16
  Constant8 : Constant  Value=C_ADC_MotorTemp1Gain_f32
  Constant9 : Constant  Value=C_ADC_IGBTTempGain_f32
  Product{,1..14} (15 alike) : Product
  GainParam : Outport
  wires:
  Constant/1 -> Product/1
  Constant1/1 -> Product/2
  Product/1 -> Bus Creator/1  "IaGain"
  Constant3/1 -> Product1/2
  Constant2/1 -> Product1/1
  Constant5/1 -> Product2/2
  Constant4/1 -> Product2/1
  Product1/1 -> Bus Creator/2  "IbGain"
  Product2/1 -> Bus Creator/3  "IcGain"
  Bus Creator/1 -> GainParam/1
  Constant7/1 -> Product3/2
  Product3/1 -> Bus Creator/4  "UdcGain"
  Constant8/1 -> Product4/1
  Constant10/1 -> Product5/1
  Constant11/1 -> Product6/1
  Constant12/1 -> Product7/1
  Constant14/1 -> Product8/1
  Constant13/1 -> Product4/2
  Constant9/1 -> Product9/1
  Constant15/1 -> Product9/2
  Constant16/1 -> Product5/2
  Constant17/1 -> Product6/2
  Constant18/1 -> Product7/2
  Constant19/1 -> Product8/2
  Product4/1 -> Bus Creator/5  "MotorTempGain"
  Product9/1 -> Bus Creator/6  "IGBTTempGain"
  Product5/1 -> Bus Creator/7  "P5VGain"
  Product6/1 -> Bus Creator/8  "P12VGain"
  Product7/1 -> Bus Creator/9  "P15VGain"
  Product8/1 -> Bus Creator/10  "Acc1Gain"
  Constant20/1 -> Product10/1
  Constant21/1 -> Product10/2
  Product10/1 -> Bus Creator/11  "IdcGain"
  Constant23/1 -> Product11/2
  Product11/1 -> Bus Creator/12  "HSTempGain"
  Constant24/1 -> Product12/1
  Constant25/1 -> Product12/2
  Product12/1 -> Bus Creator/13  "BrakeGain"
  Constant26/1 -> Product13/1
  Constant27/1 -> Product14/1
  Constant28/1 -> Product13/2
  Constant29/1 -> Product14/2
  Product13/1 -> Bus Creator/14  "VKeyGain"
  Product14/1 -> Bus Creator/15  "HalfVdcGain"
  Constant6/1 -> Product3/1
  Constant22/1 -> Product11/1

== system MCU_Input/Input_10ms/ADC_10ms/OffsetInit ==
  Bus Creator : BusCreator  Inputs=12
  Constant : Constant  Value=ParamCfg_UdcDefValue_u16
  Constant1 : Constant  Value=C_ADC_Acc1Offset_i32  OutDataTypeStr=int32
  Constant10 : Constant  Value=ParamCfg_UdcDefValue_u16  OutDataTypeStr=int32
  Constant11 : Constant  Value=ParamCfg_UdcDefValue_u16  OutDataTypeStr=int32
  Constant2 : Constant  Value=C_ADC_MotorTemp1Offset_i32  OutDataTypeStr=int32
  Constant3 : Constant  Value=C_ADC_P5VOffset_i32  OutDataTypeStr=int32
  Constant4 : Constant  Value=C_ADC_P12VOffset_i32  OutDataTypeStr=int32
  Constant5 : Constant  Value=C_ADC_P15VOffset_i32  OutDataTypeStr=int32
  Constant6 : Constant  Value=C_ADC_IGBTTempOffset_i32  OutDataTypeStr=int32
  Constant7 : Constant  Value=C_ADC_IdcOffset_i32  OutDataTypeStr=int32
  Constant8 : Constant  Value=C_ADC_HSTempOffset_i32  OutDataTypeStr=int32
  Constant9 : Constant  Value=C_ADC_BrakeOffset_i32  OutDataTypeStr=int32
  OffsetParam : Outport
  wires:
  Bus Creator/1 -> OffsetParam/1
  Constant/1 -> Bus Creator/1  "UdcOffset"
  Constant1/1 -> Bus Creator/2  "Acc1Offset"
  Constant2/1 -> Bus Creator/3  "MotorTemp1Offset"
  Constant3/1 -> Bus Creator/4  "P5VOffset"
  Constant4/1 -> Bus Creator/5  "P12VOffset"
  Constant5/1 -> Bus Creator/6  "P15VOffset"
  Constant6/1 -> Bus Creator/7  "IGBTTempOffset"
  Constant7/1 -> Bus Creator/8  "IdcOffset"
  Constant8/1 -> Bus Creator/9  "HSTempOffset"
  Constant9/1 -> Bus Creator/10  "BrakeOffset"
  Constant10/1 -> Bus Creator/11  "VKeyOffset"
  Constant11/1 -> Bus Creator/12  "HalfVdcOffset"

== system MCU_Input/Input_10ms/GPIO_Get_10ms/Read ==
  Enable : EnablePort
  Function Caller : FunctionCaller  FunctionPrototype=OriginalSignal = GPIOInput_DGI_FD_b()  InputArgumentSpecifications=<Enter example>  OutputArgumentSpecifications=uint16(1)
  Function Caller1 : FunctionCaller  FunctionPrototype=OriginalSignal = GPIOInput_DGI_XH_b()  InputArgumentSpecifications=<Enter example>  OutputArgumentSpecifications=uint16(1)
  Function Caller2 : FunctionCaller  FunctionPrototype=OriginalSignal = GPIOInput_DGI_ABS_b()  InputArgumentSpecifications=<Enter example>  OutputArgumentSpecifications=uint16(1)
  Function Caller3 : FunctionCaller  FunctionPrototype=OriginalSignal = GPIOInput_DGI_DP_b()  InputArgumentSpecifications=<Enter example>  OutputArgumentSpecifications=uint16(1)
  Function Caller4 : FunctionCaller  FunctionPrototype=OriginalSignal = GPIOInput_DGI_DC_b()  InputArgumentSpecifications=<Enter example>  OutputArgumentSpecifications=uint16(1)
  Function Caller5 : FunctionCaller  FunctionPrototype=OriginalSignal = GPIOInput_DGI_SG1_b()  InputArgumentSpecifications=<Enter example>  OutputArgumentSpecifications=uint16(1)
  Function Caller6 : FunctionCaller  FunctionPrototype=OriginalSignal = GPIOInput_DGI_SG2_b()  InputArgumentSpecifications=<Enter example>  OutputArgumentSpecifications=uint16(1)
  Function Caller7 : FunctionCaller  FunctionPrototype=OriginalSignal = GPIOInput_DGI_DW_b()  InputArgumentSpecifications=<Enter example>  OutputArgumentSpecifications=uint16(1)
  Function Caller8 : FunctionCaller  FunctionPrototype=OriginalSignal = GPIOInput_DGI_BKL_b()  InputArgumentSpecifications=<Enter example>  OutputArgumentSpecifications=uint16(1)
  GPIO_Signal_filter : Subsystem
  Gpio_AntiTheftSignal : Outport
  Gpio_RepairSignal : Outport  Port=2
  Gpio_ABSSignal : Outport  Port=3
  Gpio_HDCSignal : Outport  Port=4
  Gpio_BackSignal : Outport  Port=5
  Gpio_CCSSignal : Outport  Port=6
  Gpio_SportSignal : Outport  Port=7
  Gpio_KGearSignal : Outport  Port=8
  Gpio_BrakeSignal : Outport  Port=9
  wires:
  GPIO_Signal_filter/1(AntiTheftSignal) -> Gpio_AntiTheftSignal/1
  GPIO_Signal_filter/2(RepairSignal) -> Gpio_RepairSignal/1
  GPIO_Signal_filter/3(ABSSignal) -> Gpio_ABSSignal/1
  GPIO_Signal_filter/4(HDCSignal) -> Gpio_HDCSignal/1
  GPIO_Signal_filter/5(BackSignal) -> Gpio_BackSignal/1
  GPIO_Signal_filter/6(CCSSignal) -> Gpio_CCSSignal/1
  GPIO_Signal_filter/7(SportSignal) -> Gpio_SportSignal/1
  GPIO_Signal_filter/8(KGearSignal) -> Gpio_KGearSignal/1
  GPIO_Signal_filter/9(BrakeSignal) -> Gpio_BrakeSignal/1
  Function Caller/1 -> GPIO_Signal_filter/1(AntiTheftOriginalSignal)  "M_GPIO_AntiTheftOriginalSignal_u16"
  Function Caller8/1 -> GPIO_Signal_filter/9(BrakeOriginalSignal)  "M_GPIO_BrakeOriginalSignal_u16"
  Function Caller1/1 -> GPIO_Signal_filter/2(RepairOriginalSignal)  "M_GPIO_RepairOriginalSignal_u16"
  Function Caller2/1 -> GPIO_Signal_filter/3(ABSOriginalSignal)  "M_GPIO_ABSOriginalSignal_u16"
  Function Caller3/1 -> GPIO_Signal_filter/4(HDCOriginalSignal)  "M_GPIO_HDCOriginalSignal_u16"
  Function Caller4/1 -> GPIO_Signal_filter/5(BackOriginalSignal)  "M_GPIO_BackOriginalSignal_u16"
  Function Caller5/1 -> GPIO_Signal_filter/6(CCSOriginalSignal)  "M_GPIO_CCSOriginalSignal_u16"
  Function Caller6/1 -> GPIO_Signal_filter/7(SportOriginalSignal)  "M_GPIO_SportOriginalSignal_u16"
  Function Caller7/1 -> GPIO_Signal_filter/8(KGearOriginalSignal)  "M_GPIO_KGearOriginalSignal_u16"
